simulink model "ddc_bpm_476_066"  (Simulink 7.8)
settings: Solver=ode45  StartTime=0.0  StopTime=4e-4  RelTol=1e-3
undefined symbols (not defined in the file): dt_sim, frev_476, Fs_adc, xlipgetpartsetting
libraries: xbsIndex_r4 x498, simulink x3
(part 2 of 5)

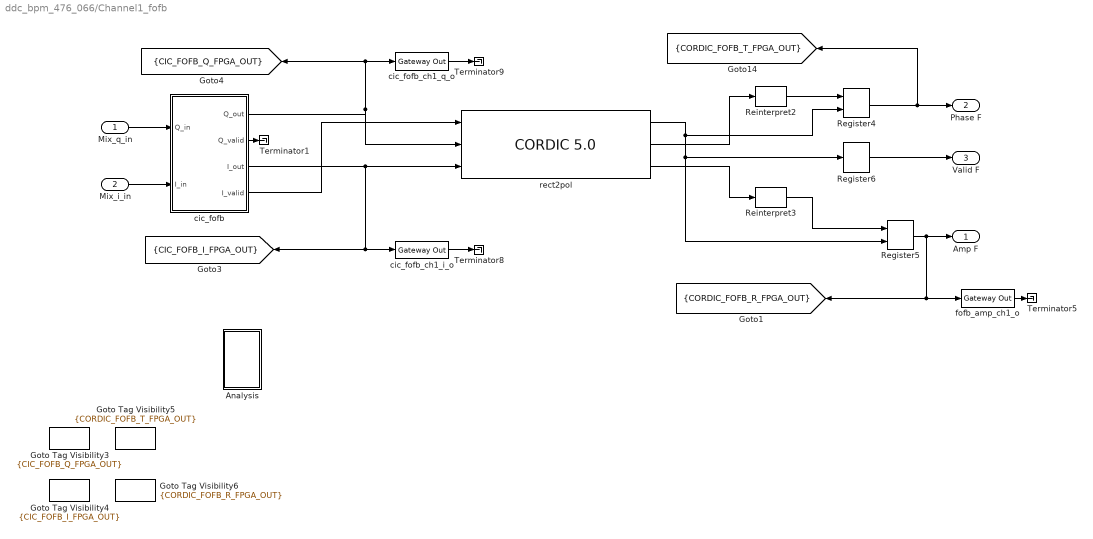
== system ddc_bpm_476_066/Channel1_fofb ==
  Mix_q_in : Inport
  Mix_i_in : Inport  Port=2
  Analysis : Subsystem
  Goto Tag Visibility3 : GotoTagVisibility  GotoTag=CIC_FOFB_Q_FPGA_OUT
  Goto Tag Visibility4 : GotoTagVisibility  GotoTag=CIC_FOFB_I_FPGA_OUT
  Goto Tag Visibility5 : GotoTagVisibility  GotoTag=CORDIC_FOFB_T_FPGA_OUT
  Goto Tag Visibility6 : GotoTagVisibility  GotoTag=CORDIC_FOFB_R_FPGA_OUT
  Register4 : xbsIndex_r4/Register  init=0  rst=off  en=on  dbl_ovrd=off  block_type=register
  Register5 : xbsIndex_r4/Register  init=0  rst=off  en=on  dbl_ovrd=off  block_type=register
  Register6 : xbsIndex_r4/Register  init=0  rst=off  en=off  dbl_ovrd=off  block_type=register
  Reinterpret2 : xbsIndex_r4/Reinterpret  force_arith_type=off  arith_type=Unsigned  force_bin_pt=off  bin_pt=18  block_type=reinterpret
  Reinterpret3 : xbsIndex_r4/Reinterpret  force_arith_type=off  arith_type=Unsigned  force_bin_pt=off  bin_pt=19  block_type=reinterpret
  Terminator{1,5,8..9} (4 alike) : Terminator
  cic_fofb : Subsystem
  cic_fofb_ch1_i_o : xbsIndex_r4/Gateway Out  inherit_from_input=on  hdl_port=on  timing_constraint=Data Rate  locs_specified=off  LOCs={}  UseAsDAC=off  DACChannel='1'  block_type=gatewayout
      settings: infoedit="Gateway out block.  Converts Xilinx fixed-point or floating-point type inputs into ouputs of type Simulink integer, single, double, or fixed point.<br><br>Hardware notes:  In hardware these blocks become top level output ports or are discarded, depending on how they are configured."
  cic_fofb_ch1_q_o : xbsIndex_r4/Gateway Out  inherit_from_input=on  hdl_port=on  timing_constraint=Data Rate  locs_specified=off  LOCs={}  UseAsDAC=off  DACChannel='1'  block_type=gatewayout
      settings: infoedit="Gateway out block.  Converts Xilinx fixed-point or floating-point type inputs into ouputs of type Simulink integer, single, double, or fixed point.<br><br>Hardware notes:  In hardware these blocks become top level output ports or are discarded, depending on how they are configured."
  fofb_amp_ch1_o : xbsIndex_r4/Gateway Out  inherit_from_input=on  hdl_port=on  timing_constraint=Data Rate  locs_specified=off  LOCs={}  UseAsDAC=off  DACChannel='1'  block_type=gatewayout
      settings: infoedit="Gateway out block.  Converts Xilinx fixed-point or floating-point type inputs into ouputs of type Simulink integer, single, double, or fixed point.<br><br>Hardware notes:  In hardware these blocks become top level output ports or are discarded, depending on how they are configured."
  rect2pol : xbsIndex_r4/CORDIC 5.0   functional_selection=Translate  architectural_configuration=Parallel  pipelining_mode=Maximum  data_format=SignedFraction  phase_format=Radians  input_width=25  output_width=25  round_mode=Nearest_Even  iterations=0  precision=0  compensation_scaling=BRAM  coarse_rotation=on  aclken=off  aresetn=off  out_tready=off  cartesian_has_tuser=off  cartesian_has_tlast=off  cartesian_tuser_width=1  phase_has_tuser=off  phase_has_tlast=off  phase_tuser_width=1  out_tlast_behv=Null  flow_control=NonBlocking  optimize_goal=Resources  trim_axipin_name=on  ip_name=CORDIC  ip_version=5.0  dsptool_ready=true  ipcore_usecache=true  ipcore_useipmodelcache=true  wrapper_available=true  port_translation_map={ 'aclken' => 'en', 'aresetn' => 'rst' }  block_type=cordic_v5_0
      settings: infoedit=CORDIC 5.0
  Amp F : Outport
  Phase F : Outport  Port=2
  Valid F : Outport  Port=3
  tag scope: CIC_FOFB_I_FPGA_OUT=scoped, CIC_FOFB_Q_FPGA_OUT=scoped, CORDIC_FOFB_R_FPGA_OUT=scoped, CORDIC_FOFB_T_FPGA_OUT=scoped
  wires:
  cic_fofb/3(I_out) -> rect2pol/3, cic_fofb_ch1_i_o/1, [CIC_FOFB_I_FPGA_OUT]
  cic_fofb/1(Q_out) -> [CIC_FOFB_Q_FPGA_OUT], cic_fofb_ch1_q_o/1, rect2pol/2
  cic_fofb/2(Q_valid) -> Terminator1/1
  rect2pol/1 -> Register4/2, Register5/2, Register6/1
  rect2pol/2 -> Reinterpret2/1
  rect2pol/3 -> Reinterpret3/1
  Register4/1 -> Phase F/1, [CORDIC_FOFB_T_FPGA_OUT]
  Register5/1 -> Amp F/1, [CORDIC_FOFB_R_FPGA_OUT], fofb_amp_ch1_o/1
  Register6/1 -> Valid F/1
  Reinterpret2/1 -> Register4/1
  Reinterpret3/1 -> Register5/1
  fofb_amp_ch1_o/1 -> Terminator5/1
  cic_fofb_ch1_q_o/1 -> Terminator9/1
  cic_fofb_ch1_i_o/1 -> Terminator8/1
  Mix_q_in/1 -> cic_fofb/1(Q_in)
  Mix_i_in/1 -> cic_fofb/2(I_in)
  cic_fofb/4(I_valid) -> rect2pol/1

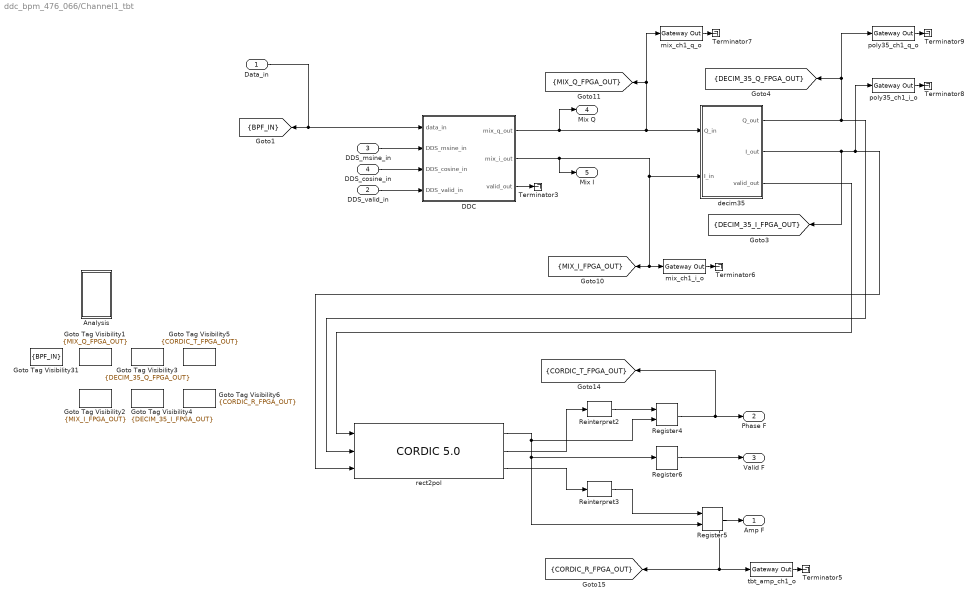
== system ddc_bpm_476_066/Channel1_tbt ==
  Data_in : Inport
  DDS_valid_in : Inport  Port=2
  DDS_msine_in : Inport  Port=3
  DDS_cosine_in : Inport  Port=4
  Analysis : Subsystem
  DDC : Subsystem
  Goto Tag Visibility1 : GotoTagVisibility  GotoTag=MIX_Q_FPGA_OUT
  Goto Tag Visibility2 : GotoTagVisibility  GotoTag=MIX_I_FPGA_OUT
  Goto Tag Visibility3 : GotoTagVisibility  GotoTag=DECIM_35_Q_FPGA_OUT
  Goto Tag Visibility31 : GotoTagVisibility  GotoTag=BPF_IN
  Goto Tag Visibility4 : GotoTagVisibility  GotoTag=DECIM_35_I_FPGA_OUT
  Goto Tag Visibility5 : GotoTagVisibility  GotoTag=CORDIC_T_FPGA_OUT
  Goto Tag Visibility6 : GotoTagVisibility  GotoTag=CORDIC_R_FPGA_OUT
  Register4 : xbsIndex_r4/Register  init=0  rst=off  en=on  dbl_ovrd=off  block_type=register
  Register5 : xbsIndex_r4/Register  init=0  rst=off  en=on  dbl_ovrd=off  block_type=register
  Register6 : xbsIndex_r4/Register  init=0  rst=off  en=off  dbl_ovrd=off  block_type=register
  Reinterpret2 : xbsIndex_r4/Reinterpret  force_arith_type=off  arith_type=Unsigned  force_bin_pt=off  bin_pt=18  block_type=reinterpret
  Reinterpret3 : xbsIndex_r4/Reinterpret  force_arith_type=off  arith_type=Unsigned  force_bin_pt=off  bin_pt=19  block_type=reinterpret
  Terminator{3,5..9} (6 alike) : Terminator
  decim35 : Subsystem
  mix_ch1_i_o : xbsIndex_r4/Gateway Out  inherit_from_input=on  hdl_port=on  timing_constraint=Data Rate  locs_specified=off  LOCs={}  UseAsDAC=off  DACChannel='1'  block_type=gatewayout
      settings: infoedit="Gateway out block.  Converts Xilinx fixed-point or floating-point type inputs into ouputs of type Simulink integer, single, double, or fixed point.<br><br>Hardware notes:  In hardware these blocks become top level output ports or are discarded, depending on how they are configured."
  mix_ch1_q_o : xbsIndex_r4/Gateway Out  inherit_from_input=on  hdl_port=on  timing_constraint=Data Rate  locs_specified=off  LOCs={}  UseAsDAC=off  DACChannel='1'  block_type=gatewayout
      settings: infoedit="Gateway out block.  Converts Xilinx fixed-point or floating-point type inputs into ouputs of type Simulink integer, single, double, or fixed point.<br><br>Hardware notes:  In hardware these blocks become top level output ports or are discarded, depending on how they are configured."
  poly35_ch1_i_o : xbsIndex_r4/Gateway Out  inherit_from_input=on  hdl_port=on  timing_constraint=Data Rate  locs_specified=off  LOCs={}  UseAsDAC=off  DACChannel='1'  block_type=gatewayout
      settings: infoedit="Gateway out block.  Converts Xilinx fixed-point or floating-point type inputs into ouputs of type Simulink integer, single, double, or fixed point.<br><br>Hardware notes:  In hardware these blocks become top level output ports or are discarded, depending on how they are configured."
  poly35_ch1_q_o : xbsIndex_r4/Gateway Out  inherit_from_input=on  hdl_port=on  timing_constraint=Data Rate  locs_specified=off  LOCs={}  UseAsDAC=off  DACChannel='1'  block_type=gatewayout
      settings: infoedit="Gateway out block.  Converts Xilinx fixed-point or floating-point type inputs into ouputs of type Simulink integer, single, double, or fixed point.<br><br>Hardware notes:  In hardware these blocks become top level output ports or are discarded, depending on how they are configured."
  rect2pol : xbsIndex_r4/CORDIC 5.0   functional_selection=Translate  architectural_configuration=Parallel  pipelining_mode=Maximum  data_format=SignedFraction  phase_format=Radians  input_width=25  output_width=25  round_mode=Nearest_Even  iterations=0  precision=0  compensation_scaling=BRAM  coarse_rotation=on  aclken=off  aresetn=off  out_tready=off  cartesian_has_tuser=off  cartesian_has_tlast=off  cartesian_tuser_width=1  phase_has_tuser=off  phase_has_tlast=off  phase_tuser_width=1  out_tlast_behv=Null  flow_control=NonBlocking  optimize_goal=Resources  trim_axipin_name=on  ip_name=CORDIC  ip_version=5.0  dsptool_ready=true  ipcore_usecache=true  ipcore_useipmodelcache=true  wrapper_available=true  port_translation_map={ 'aclken' => 'en', 'aresetn' => 'rst' }  block_type=cordic_v5_0
      settings: infoedit=CORDIC 5.0
  tbt_amp_ch1_o : xbsIndex_r4/Gateway Out  inherit_from_input=on  hdl_port=on  timing_constraint=Data Rate  locs_specified=off  LOCs={}  UseAsDAC=off  DACChannel='1'  block_type=gatewayout
      settings: infoedit="Gateway out block.  Converts Xilinx fixed-point or floating-point type inputs into ouputs of type Simulink integer, single, double, or fixed point.<br><br>Hardware notes:  In hardware these blocks become top level output ports or are discarded, depending on how they are configured."
  Amp F : Outport
  Phase F : Outport  Port=2
  Valid F : Outport  Port=3
  Mix Q : Outport  Port=4
  Mix I : Outport  Port=5
  tag scope: BPF_IN=scoped, CORDIC_R_FPGA_OUT=scoped, CORDIC_T_FPGA_OUT=scoped, DECIM_35_I_FPGA_OUT=scoped, DECIM_35_Q_FPGA_OUT=scoped, MIX_I_FPGA_OUT=scoped, MIX_Q_FPGA_OUT=scoped
  wires:
  Data_in/1 -> [BPF_IN], DDC/1(data_in)
  DDC/2(mix_i_out) -> decim35/2(I_in), [MIX_I_FPGA_OUT], mix_ch1_i_o/1, Mix I/1
  DDC/3(valid_out) -> Terminator3/1
  DDC/1(mix_q_out) -> decim35/1(Q_in), [MIX_Q_FPGA_OUT], mix_ch1_q_o/1, Mix Q/1
  decim35/2(I_out) -> [DECIM_35_I_FPGA_OUT], rect2pol/3, poly35_ch1_i_o/1
  decim35/1(Q_out) -> rect2pol/2, [DECIM_35_Q_FPGA_OUT], poly35_ch1_q_o/1
  decim35/3(valid_out) -> rect2pol/1
  rect2pol/1 -> Register4/2, Register5/2, Register6/1
  rect2pol/2 -> Reinterpret2/1
  rect2pol/3 -> Reinterpret3/1
  Register4/1 -> Phase F/1, [CORDIC_T_FPGA_OUT]
  Register5/1 -> Amp F/1, [CORDIC_R_FPGA_OUT], tbt_amp_ch1_o/1
  Register6/1 -> Valid F/1
  Reinterpret2/1 -> Register4/1
  Reinterpret3/1 -> Register5/1
  tbt_amp_ch1_o/1 -> Terminator5/1
  mix_ch1_i_o/1 -> Terminator6/1
  mix_ch1_q_o/1 -> Terminator7/1
  poly35_ch1_q_o/1 -> Terminator9/1
  poly35_ch1_i_o/1 -> Terminator8/1
  DDS_valid_in/1 -> DDC/4(DDS_valid_in)
  DDS_msine_in/1 -> DDC/2(DDS_msine_in)
  DDS_cosine_in/1 -> DDC/3(DDS_cosine_in)

== system ddc_bpm_476_066/Channel2_fofb ==
  Mix_q_in : Inport
  Mix_i_in : Inport  Port=2
  Analysis : Subsystem
  Goto Tag Visibility3 : GotoTagVisibility  GotoTag=CIC_FOFB_Q_FPGA_OUT
  Goto Tag Visibility4 : GotoTagVisibility  GotoTag=CIC_FOFB_I_FPGA_OUT
  Goto Tag Visibility5 : GotoTagVisibility  GotoTag=CORDIC_FOFB_T_FPGA_OUT
  Goto Tag Visibility6 : GotoTagVisibility  GotoTag=CORDIC_FOFB_R_FPGA_OUT
  Register4 : xbsIndex_r4/Register  init=0  rst=off  en=on  dbl_ovrd=off  block_type=register
  Register5 : xbsIndex_r4/Register  init=0  rst=off  en=on  dbl_ovrd=off  block_type=register
  Register6 : xbsIndex_r4/Register  init=0  rst=off  en=off  dbl_ovrd=off  block_type=register
  Reinterpret2 : xbsIndex_r4/Reinterpret  force_arith_type=off  arith_type=Unsigned  force_bin_pt=off  bin_pt=18  block_type=reinterpret
  Reinterpret3 : xbsIndex_r4/Reinterpret  force_arith_type=off  arith_type=Unsigned  force_bin_pt=off  bin_pt=19  block_type=reinterpret
  Terminator{1,5,8..9} (4 alike) : Terminator
  cic_fofb : Subsystem
  cic_fofb_ch2_i_o : xbsIndex_r4/Gateway Out  inherit_from_input=on  hdl_port=on  timing_constraint=Data Rate  locs_specified=off  LOCs={}  UseAsDAC=off  DACChannel='1'  block_type=gatewayout
      settings: infoedit="Gateway out block.  Converts Xilinx fixed-point or floating-point type inputs into ouputs of type Simulink integer, single, double, or fixed point.<br><br>Hardware notes:  In hardware these blocks become top level output ports or are discarded, depending on how they are configured."
  cic_fofb_ch2_q_o : xbsIndex_r4/Gateway Out  inherit_from_input=on  hdl_port=on  timing_constraint=Data Rate  locs_specified=off  LOCs={}  UseAsDAC=off  DACChannel='1'  block_type=gatewayout
      settings: infoedit="Gateway out block.  Converts Xilinx fixed-point or floating-point type inputs into ouputs of type Simulink integer, single, double, or fixed point.<br><br>Hardware notes:  In hardware these blocks become top level output ports or are discarded, depending on how they are configured."
  fofb_amp_ch2_o : xbsIndex_r4/Gateway Out  inherit_from_input=on  hdl_port=on  timing_constraint=Data Rate  locs_specified=off  LOCs={}  UseAsDAC=off  DACChannel='1'  block_type=gatewayout
      settings: infoedit="Gateway out block.  Converts Xilinx fixed-point or floating-point type inputs into ouputs of type Simulink integer, single, double, or fixed point.<br><br>Hardware notes:  In hardware these blocks become top level output ports or are discarded, depending on how they are configured."
  rect2pol : xbsIndex_r4/CORDIC 5.0   functional_selection=Translate  architectural_configuration=Parallel  pipelining_mode=Maximum  data_format=SignedFraction  phase_format=Radians  input_width=25  output_width=25  round_mode=Nearest_Even  iterations=0  precision=0  compensation_scaling=BRAM  coarse_rotation=on  aclken=off  aresetn=off  out_tready=off  cartesian_has_tuser=off  cartesian_has_tlast=off  cartesian_tuser_width=1  phase_has_tuser=off  phase_has_tlast=off  phase_tuser_width=1  out_tlast_behv=Null  flow_control=NonBlocking  optimize_goal=Resources  trim_axipin_name=on  ip_name=CORDIC  ip_version=5.0  dsptool_ready=true  ipcore_usecache=true  ipcore_useipmodelcache=true  wrapper_available=true  port_translation_map={ 'aclken' => 'en', 'aresetn' => 'rst' }  block_type=cordic_v5_0
      settings: infoedit=CORDIC 5.0
  Amp F : Outport
  Phase F : Outport  Port=2
  Valid F : Outport  Port=3
  tag scope: CIC_FOFB_I_FPGA_OUT=scoped, CIC_FOFB_Q_FPGA_OUT=scoped, CORDIC_FOFB_R_FPGA_OUT=scoped, CORDIC_FOFB_T_FPGA_OUT=scoped
  wires:
  cic_fofb/3(I_out) -> rect2pol/3, cic_fofb_ch2_i_o/1, [CIC_FOFB_I_FPGA_OUT]
  cic_fofb/1(Q_out) -> [CIC_FOFB_Q_FPGA_OUT], cic_fofb_ch2_q_o/1, rect2pol/2
  cic_fofb/2(Q_valid) -> Terminator1/1
  rect2pol/1 -> Register4/2, Register5/2, Register6/1
  rect2pol/2 -> Reinterpret2/1
  rect2pol/3 -> Reinterpret3/1
  Register4/1 -> Phase F/1, [CORDIC_FOFB_T_FPGA_OUT]
  Register5/1 -> Amp F/1, [CORDIC_FOFB_R_FPGA_OUT], fofb_amp_ch2_o/1
  Register6/1 -> Valid F/1
  Reinterpret2/1 -> Register4/1
  Reinterpret3/1 -> Register5/1
  fofb_amp_ch2_o/1 -> Terminator5/1
  cic_fofb_ch2_q_o/1 -> Terminator9/1
  cic_fofb_ch2_i_o/1 -> Terminator8/1
  Mix_q_in/1 -> cic_fofb/1(Q_in)
  Mix_i_in/1 -> cic_fofb/2(I_in)
  cic_fofb/4(I_valid) -> rect2pol/1

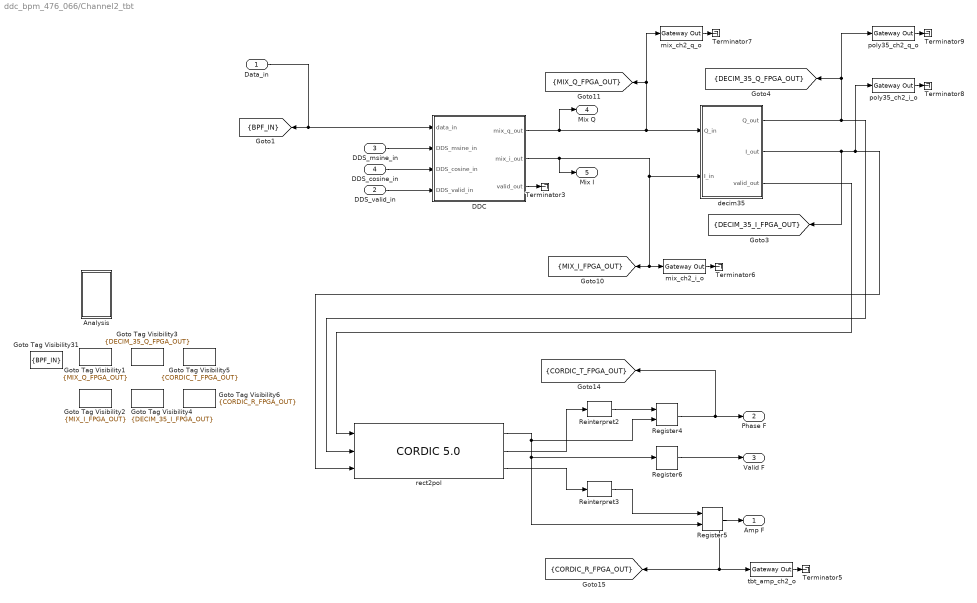
== system ddc_bpm_476_066/Channel2_tbt ==
  Data_in : Inport
  DDS_valid_in : Inport  Port=2
  DDS_msine_in : Inport  Port=3
  DDS_cosine_in : Inport  Port=4
  Analysis : Subsystem
  DDC : Subsystem
  Goto Tag Visibility1 : GotoTagVisibility  GotoTag=MIX_Q_FPGA_OUT
  Goto Tag Visibility2 : GotoTagVisibility  GotoTag=MIX_I_FPGA_OUT
  Goto Tag Visibility3 : GotoTagVisibility  GotoTag=DECIM_35_Q_FPGA_OUT
  Goto Tag Visibility31 : GotoTagVisibility  GotoTag=BPF_IN
  Goto Tag Visibility4 : GotoTagVisibility  GotoTag=DECIM_35_I_FPGA_OUT
  Goto Tag Visibility5 : GotoTagVisibility  GotoTag=CORDIC_T_FPGA_OUT
  Goto Tag Visibility6 : GotoTagVisibility  GotoTag=CORDIC_R_FPGA_OUT
  Register4 : xbsIndex_r4/Register  init=0  rst=off  en=on  dbl_ovrd=off  block_type=register
  Register5 : xbsIndex_r4/Register  init=0  rst=off  en=on  dbl_ovrd=off  block_type=register
  Register6 : xbsIndex_r4/Register  init=0  rst=off  en=off  dbl_ovrd=off  block_type=register
  Reinterpret2 : xbsIndex_r4/Reinterpret  force_arith_type=off  arith_type=Unsigned  force_bin_pt=off  bin_pt=18  block_type=reinterpret
  Reinterpret3 : xbsIndex_r4/Reinterpret  force_arith_type=off  arith_type=Unsigned  force_bin_pt=off  bin_pt=19  block_type=reinterpret
  Terminator{3,5..9} (6 alike) : Terminator
  decim35 : Subsystem
  mix_ch2_i_o : xbsIndex_r4/Gateway Out  inherit_from_input=on  hdl_port=on  timing_constraint=Data Rate  locs_specified=off  LOCs={}  UseAsDAC=off  DACChannel='1'  block_type=gatewayout
      settings: infoedit="Gateway out block.  Converts Xilinx fixed-point or floating-point type inputs into ouputs of type Simulink integer, single, double, or fixed point.<br><br>Hardware notes:  In hardware these blocks become top level output ports or are discarded, depending on how they are configured."
  mix_ch2_q_o : xbsIndex_r4/Gateway Out  inherit_from_input=on  hdl_port=on  timing_constraint=Data Rate  locs_specified=off  LOCs={}  UseAsDAC=off  DACChannel='1'  block_type=gatewayout
      settings: infoedit="Gateway out block.  Converts Xilinx fixed-point or floating-point type inputs into ouputs of type Simulink integer, single, double, or fixed point.<br><br>Hardware notes:  In hardware these blocks become top level output ports or are discarded, depending on how they are configured."
  poly35_ch2_i_o : xbsIndex_r4/Gateway Out  inherit_from_input=on  hdl_port=on  timing_constraint=Data Rate  locs_specified=off  LOCs={}  UseAsDAC=off  DACChannel='1'  block_type=gatewayout
      settings: infoedit="Gateway out block.  Converts Xilinx fixed-point or floating-point type inputs into ouputs of type Simulink integer, single, double, or fixed point.<br><br>Hardware notes:  In hardware these blocks become top level output ports or are discarded, depending on how they are configured."
  poly35_ch2_q_o : xbsIndex_r4/Gateway Out  inherit_from_input=on  hdl_port=on  timing_constraint=Data Rate  locs_specified=off  LOCs={}  UseAsDAC=off  DACChannel='1'  block_type=gatewayout
      settings: infoedit="Gateway out block.  Converts Xilinx fixed-point or floating-point type inputs into ouputs of type Simulink integer, single, double, or fixed point.<br><br>Hardware notes:  In hardware these blocks become top level output ports or are discarded, depending on how they are configured."
  rect2pol : xbsIndex_r4/CORDIC 5.0   functional_selection=Translate  architectural_configuration=Parallel  pipelining_mode=Maximum  data_format=SignedFraction  phase_format=Radians  input_width=25  output_width=25  round_mode=Nearest_Even  iterations=0  precision=0  compensation_scaling=BRAM  coarse_rotation=on  aclken=off  aresetn=off  out_tready=off  cartesian_has_tuser=off  cartesian_has_tlast=off  cartesian_tuser_width=1  phase_has_tuser=off  phase_has_tlast=off  phase_tuser_width=1  out_tlast_behv=Null  flow_control=NonBlocking  optimize_goal=Resources  trim_axipin_name=on  ip_name=CORDIC  ip_version=5.0  dsptool_ready=true  ipcore_usecache=true  ipcore_useipmodelcache=true  wrapper_available=true  port_translation_map={ 'aclken' => 'en', 'aresetn' => 'rst' }  block_type=cordic_v5_0
      settings: infoedit=CORDIC 5.0
  tbt_amp_ch2_o : xbsIndex_r4/Gateway Out  inherit_from_input=on  hdl_port=on  timing_constraint=Data Rate  locs_specified=off  LOCs={}  UseAsDAC=off  DACChannel='1'  block_type=gatewayout
      settings: infoedit="Gateway out block.  Converts Xilinx fixed-point or floating-point type inputs into ouputs of type Simulink integer, single, double, or fixed point.<br><br>Hardware notes:  In hardware these blocks become top level output ports or are discarded, depending on how they are configured."
  Amp F : Outport
  Phase F : Outport  Port=2
  Valid F : Outport  Port=3
  Mix Q : Outport  Port=4
  Mix I : Outport  Port=5
  tag scope: BPF_IN=scoped, CORDIC_R_FPGA_OUT=scoped, CORDIC_T_FPGA_OUT=scoped, DECIM_35_I_FPGA_OUT=scoped, DECIM_35_Q_FPGA_OUT=scoped, MIX_I_FPGA_OUT=scoped, MIX_Q_FPGA_OUT=scoped
  wires:
  Data_in/1 -> [BPF_IN], DDC/1(data_in)
  DDC/2(mix_i_out) -> decim35/2(I_in), [MIX_I_FPGA_OUT], mix_ch2_i_o/1, Mix I/1
  DDC/3(valid_out) -> Terminator3/1
  DDC/1(mix_q_out) -> decim35/1(Q_in), [MIX_Q_FPGA_OUT], mix_ch2_q_o/1, Mix Q/1
  decim35/2(I_out) -> [DECIM_35_I_FPGA_OUT], rect2pol/3, poly35_ch2_i_o/1
  decim35/1(Q_out) -> rect2pol/2, [DECIM_35_Q_FPGA_OUT], poly35_ch2_q_o/1
  decim35/3(valid_out) -> rect2pol/1
  rect2pol/1 -> Register4/2, Register5/2, Register6/1
  rect2pol/2 -> Reinterpret2/1
  rect2pol/3 -> Reinterpret3/1
  Register4/1 -> Phase F/1, [CORDIC_T_FPGA_OUT]
  Register5/1 -> Amp F/1, [CORDIC_R_FPGA_OUT], tbt_amp_ch2_o/1
  Register6/1 -> Valid F/1
  Reinterpret2/1 -> Register4/1
  Reinterpret3/1 -> Register5/1
  tbt_amp_ch2_o/1 -> Terminator5/1
  mix_ch2_i_o/1 -> Terminator6/1
  mix_ch2_q_o/1 -> Terminator7/1
  poly35_ch2_q_o/1 -> Terminator9/1
  poly35_ch2_i_o/1 -> Terminator8/1
  DDS_valid_in/1 -> DDC/4(DDS_valid_in)
  DDS_msine_in/1 -> DDC/2(DDS_msine_in)
  DDS_cosine_in/1 -> DDC/3(DDS_cosine_in)

== system ddc_bpm_476_066/Channel3_fofb ==
  Mix_q_in : Inport
  Mix_i_in : Inport  Port=2
  Analysis : Subsystem
  Goto Tag Visibility3 : GotoTagVisibility  GotoTag=CIC_FOFB_Q_FPGA_OUT
  Goto Tag Visibility4 : GotoTagVisibility  GotoTag=CIC_FOFB_I_FPGA_OUT
  Goto Tag Visibility5 : GotoTagVisibility  GotoTag=CORDIC_FOFB_T_FPGA_OUT
  Goto Tag Visibility6 : GotoTagVisibility  GotoTag=CORDIC_FOFB_R_FPGA_OUT
  Register4 : xbsIndex_r4/Register  init=0  rst=off  en=on  dbl_ovrd=off  block_type=register
  Register5 : xbsIndex_r4/Register  init=0  rst=off  en=on  dbl_ovrd=off  block_type=register
  Register6 : xbsIndex_r4/Register  init=0  rst=off  en=off  dbl_ovrd=off  block_type=register
  Reinterpret2 : xbsIndex_r4/Reinterpret  force_arith_type=off  arith_type=Unsigned  force_bin_pt=off  bin_pt=18  block_type=reinterpret
  Reinterpret3 : xbsIndex_r4/Reinterpret  force_arith_type=off  arith_type=Unsigned  force_bin_pt=off  bin_pt=19  block_type=reinterpret
  Terminator{1,5,8..9} (4 alike) : Terminator
  cic_fofb : Subsystem
  cic_fofb_ch3_i_o : xbsIndex_r4/Gateway Out  inherit_from_input=on  hdl_port=on  timing_constraint=Data Rate  locs_specified=off  LOCs={}  UseAsDAC=off  DACChannel='1'  block_type=gatewayout
      settings: infoedit="Gateway out block.  Converts Xilinx fixed-point or floating-point type inputs into ouputs of type Simulink integer, single, double, or fixed point.<br><br>Hardware notes:  In hardware these blocks become top level output ports or are discarded, depending on how they are configured."
  cic_fofb_ch3_q_o : xbsIndex_r4/Gateway Out  inherit_from_input=on  hdl_port=on  timing_constraint=Data Rate  locs_specified=off  LOCs={}  UseAsDAC=off  DACChannel='1'  block_type=gatewayout
      settings: infoedit="Gateway out block.  Converts Xilinx fixed-point or floating-point type inputs into ouputs of type Simulink integer, single, double, or fixed point.<br><br>Hardware notes:  In hardware these blocks become top level output ports or are discarded, depending on how they are configured."
  fofb_amp_ch3_o : xbsIndex_r4/Gateway Out  inherit_from_input=on  hdl_port=on  timing_constraint=Data Rate  locs_specified=off  LOCs={}  UseAsDAC=off  DACChannel='1'  block_type=gatewayout
      settings: infoedit="Gateway out block.  Converts Xilinx fixed-point or floating-point type inputs into ouputs of type Simulink integer, single, double, or fixed point.<br><br>Hardware notes:  In hardware these blocks become top level output ports or are discarded, depending on how they are configured."
  rect2pol : xbsIndex_r4/CORDIC 5.0   functional_selection=Translate  architectural_configuration=Parallel  pipelining_mode=Maximum  data_format=SignedFraction  phase_format=Radians  input_width=25  output_width=25  round_mode=Nearest_Even  iterations=0  precision=0  compensation_scaling=BRAM  coarse_rotation=on  aclken=off  aresetn=off  out_tready=off  cartesian_has_tuser=off  cartesian_has_tlast=off  cartesian_tuser_width=1  phase_has_tuser=off  phase_has_tlast=off  phase_tuser_width=1  out_tlast_behv=Null  flow_control=NonBlocking  optimize_goal=Resources  trim_axipin_name=on  ip_name=CORDIC  ip_version=5.0  dsptool_ready=true  ipcore_usecache=true  ipcore_useipmodelcache=true  wrapper_available=true  port_translation_map={ 'aclken' => 'en', 'aresetn' => 'rst' }  block_type=cordic_v5_0
      settings: infoedit=CORDIC 5.0
  Amp F : Outport
  Phase F : Outport  Port=2
  Valid F : Outport  Port=3
  tag scope: CIC_FOFB_I_FPGA_OUT=scoped, CIC_FOFB_Q_FPGA_OUT=scoped, CORDIC_FOFB_R_FPGA_OUT=scoped, CORDIC_FOFB_T_FPGA_OUT=scoped
  wires:
  cic_fofb/3(I_out) -> rect2pol/3, cic_fofb_ch3_i_o/1, [CIC_FOFB_I_FPGA_OUT]
  cic_fofb/1(Q_out) -> [CIC_FOFB_Q_FPGA_OUT], cic_fofb_ch3_q_o/1, rect2pol/2
  cic_fofb/2(Q_valid) -> Terminator1/1
  rect2pol/1 -> Register4/2, Register5/2, Register6/1
  rect2pol/2 -> Reinterpret2/1
  rect2pol/3 -> Reinterpret3/1
  Register4/1 -> Phase F/1, [CORDIC_FOFB_T_FPGA_OUT]
  Register5/1 -> Amp F/1, [CORDIC_FOFB_R_FPGA_OUT], fofb_amp_ch3_o/1
  Register6/1 -> Valid F/1
  Reinterpret2/1 -> Register4/1
  Reinterpret3/1 -> Register5/1
  fofb_amp_ch3_o/1 -> Terminator5/1
  cic_fofb_ch3_q_o/1 -> Terminator9/1
  cic_fofb_ch3_i_o/1 -> Terminator8/1
  Mix_q_in/1 -> cic_fofb/1(Q_in)
  Mix_i_in/1 -> cic_fofb/2(I_in)
  cic_fofb/4(I_valid) -> rect2pol/1

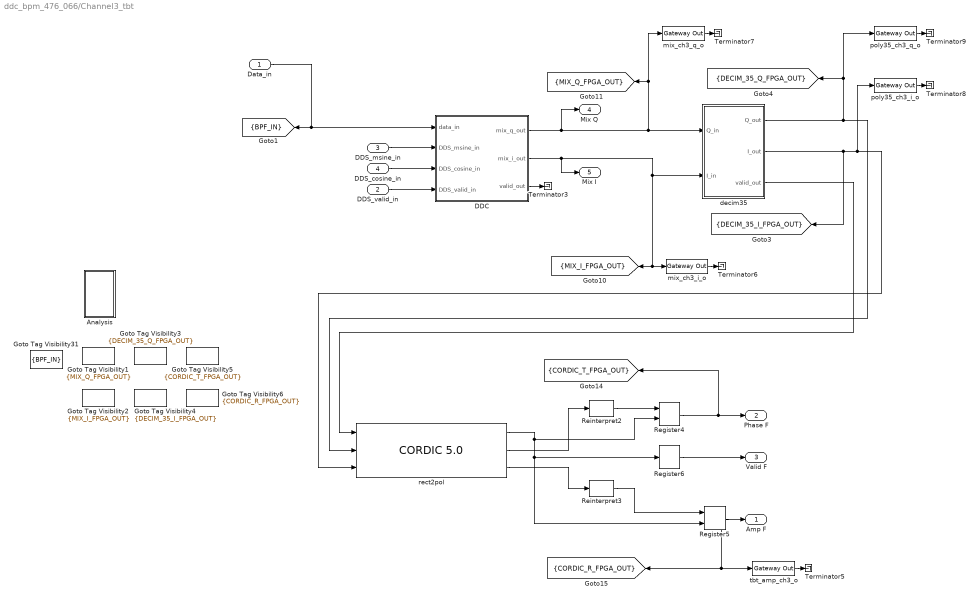
== system ddc_bpm_476_066/Channel3_tbt ==
  Data_in : Inport
  DDS_valid_in : Inport  Port=2
  DDS_msine_in : Inport  Port=3
  DDS_cosine_in : Inport  Port=4
  Analysis : Subsystem
  DDC : Subsystem
  Goto Tag Visibility1 : GotoTagVisibility  GotoTag=MIX_Q_FPGA_OUT
  Goto Tag Visibility2 : GotoTagVisibility  GotoTag=MIX_I_FPGA_OUT
  Goto Tag Visibility3 : GotoTagVisibility  GotoTag=DECIM_35_Q_FPGA_OUT
  Goto Tag Visibility31 : GotoTagVisibility  GotoTag=BPF_IN
  Goto Tag Visibility4 : GotoTagVisibility  GotoTag=DECIM_35_I_FPGA_OUT
  Goto Tag Visibility5 : GotoTagVisibility  GotoTag=CORDIC_T_FPGA_OUT
  Goto Tag Visibility6 : GotoTagVisibility  GotoTag=CORDIC_R_FPGA_OUT
  Register4 : xbsIndex_r4/Register  init=0  rst=off  en=on  dbl_ovrd=off  block_type=register
  Register5 : xbsIndex_r4/Register  init=0  rst=off  en=on  dbl_ovrd=off  block_type=register
  Register6 : xbsIndex_r4/Register  init=0  rst=off  en=off  dbl_ovrd=off  block_type=register
  Reinterpret2 : xbsIndex_r4/Reinterpret  force_arith_type=off  arith_type=Unsigned  force_bin_pt=off  bin_pt=18  block_type=reinterpret
  Reinterpret3 : xbsIndex_r4/Reinterpret  force_arith_type=off  arith_type=Unsigned  force_bin_pt=off  bin_pt=19  block_type=reinterpret
  Terminator{3,5..9} (6 alike) : Terminator
  decim35 : Subsystem
  mix_ch3_i_o : xbsIndex_r4/Gateway Out  inherit_from_input=on  hdl_port=on  timing_constraint=Data Rate  locs_specified=off  LOCs={}  UseAsDAC=off  DACChannel='1'  block_type=gatewayout
      settings: infoedit="Gateway out block.  Converts Xilinx fixed-point or floating-point type inputs into ouputs of type Simulink integer, single, double, or fixed point.<br><br>Hardware notes:  In hardware these blocks become top level output ports or are discarded, depending on how they are configured."
  mix_ch3_q_o : xbsIndex_r4/Gateway Out  inherit_from_input=on  hdl_port=on  timing_constraint=Data Rate  locs_specified=off  LOCs={}  UseAsDAC=off  DACChannel='1'  block_type=gatewayout
      settings: infoedit="Gateway out block.  Converts Xilinx fixed-point or floating-point type inputs into ouputs of type Simulink integer, single, double, or fixed point.<br><br>Hardware notes:  In hardware these blocks become top level output ports or are discarded, depending on how they are configured."
  poly35_ch3_i_o : xbsIndex_r4/Gateway Out  inherit_from_input=on  hdl_port=on  timing_constraint=Data Rate  locs_specified=off  LOCs={}  UseAsDAC=off  DACChannel='1'  block_type=gatewayout
      settings: infoedit="Gateway out block.  Converts Xilinx fixed-point or floating-point type inputs into ouputs of type Simulink integer, single, double, or fixed point.<br><br>Hardware notes:  In hardware these blocks become top level output ports or are discarded, depending on how they are configured."
  poly35_ch3_q_o : xbsIndex_r4/Gateway Out  inherit_from_input=on  hdl_port=on  timing_constraint=Data Rate  locs_specified=off  LOCs={}  UseAsDAC=off  DACChannel='1'  block_type=gatewayout
      settings: infoedit="Gateway out block.  Converts Xilinx fixed-point or floating-point type inputs into ouputs of type Simulink integer, single, double, or fixed point.<br><br>Hardware notes:  In hardware these blocks become top level output ports or are discarded, depending on how they are configured."
  rect2pol : xbsIndex_r4/CORDIC 5.0   functional_selection=Translate  architectural_configuration=Parallel  pipelining_mode=Maximum  data_format=SignedFraction  phase_format=Radians  input_width=25  output_width=25  round_mode=Nearest_Even  iterations=0  precision=0  compensation_scaling=BRAM  coarse_rotation=on  aclken=off  aresetn=off  out_tready=off  cartesian_has_tuser=off  cartesian_has_tlast=off  cartesian_tuser_width=1  phase_has_tuser=off  phase_has_tlast=off  phase_tuser_width=1  out_tlast_behv=Null  flow_control=NonBlocking  optimize_goal=Resources  trim_axipin_name=on  ip_name=CORDIC  ip_version=5.0  dsptool_ready=true  ipcore_usecache=true  ipcore_useipmodelcache=true  wrapper_available=true  port_translation_map={ 'aclken' => 'en', 'aresetn' => 'rst' }  block_type=cordic_v5_0
      settings: infoedit=CORDIC 5.0
  tbt_amp_ch3_o : xbsIndex_r4/Gateway Out  inherit_from_input=on  hdl_port=on  timing_constraint=Data Rate  locs_specified=off  LOCs={}  UseAsDAC=off  DACChannel='1'  block_type=gatewayout
      settings: infoedit="Gateway out block.  Converts Xilinx fixed-point or floating-point type inputs into ouputs of type Simulink integer, single, double, or fixed point.<br><br>Hardware notes:  In hardware these blocks become top level output ports or are discarded, depending on how they are configured."
  Amp F : Outport
  Phase F : Outport  Port=2
  Valid F : Outport  Port=3
  Mix Q : Outport  Port=4
  Mix I : Outport  Port=5
  tag scope: BPF_IN=scoped, CORDIC_R_FPGA_OUT=scoped, CORDIC_T_FPGA_OUT=scoped, DECIM_35_I_FPGA_OUT=scoped, DECIM_35_Q_FPGA_OUT=scoped, MIX_I_FPGA_OUT=scoped, MIX_Q_FPGA_OUT=scoped
  wires:
  Data_in/1 -> [BPF_IN], DDC/1(data_in)
  DDC/2(mix_i_out) -> decim35/2(I_in), [MIX_I_FPGA_OUT], mix_ch3_i_o/1, Mix I/1
  DDC/3(valid_out) -> Terminator3/1
  DDC/1(mix_q_out) -> decim35/1(Q_in), [MIX_Q_FPGA_OUT], mix_ch3_q_o/1, Mix Q/1
  decim35/2(I_out) -> [DECIM_35_I_FPGA_OUT], rect2pol/3, poly35_ch3_i_o/1
  decim35/1(Q_out) -> rect2pol/2, [DECIM_35_Q_FPGA_OUT], poly35_ch3_q_o/1
  decim35/3(valid_out) -> rect2pol/1
  rect2pol/1 -> Register4/2, Register5/2, Register6/1
  rect2pol/2 -> Reinterpret2/1
  rect2pol/3 -> Reinterpret3/1
  Register4/1 -> Phase F/1, [CORDIC_T_FPGA_OUT]
  Register5/1 -> Amp F/1, [CORDIC_R_FPGA_OUT], tbt_amp_ch3_o/1
  Register6/1 -> Valid F/1
  Reinterpret2/1 -> Register4/1
  Reinterpret3/1 -> Register5/1
  tbt_amp_ch3_o/1 -> Terminator5/1
  mix_ch3_i_o/1 -> Terminator6/1
  mix_ch3_q_o/1 -> Terminator7/1
  poly35_ch3_q_o/1 -> Terminator9/1
  poly35_ch3_i_o/1 -> Terminator8/1
  DDS_valid_in/1 -> DDC/4(DDS_valid_in)
  DDS_msine_in/1 -> DDC/2(DDS_msine_in)
  DDS_cosine_in/1 -> DDC/3(DDS_cosine_in)

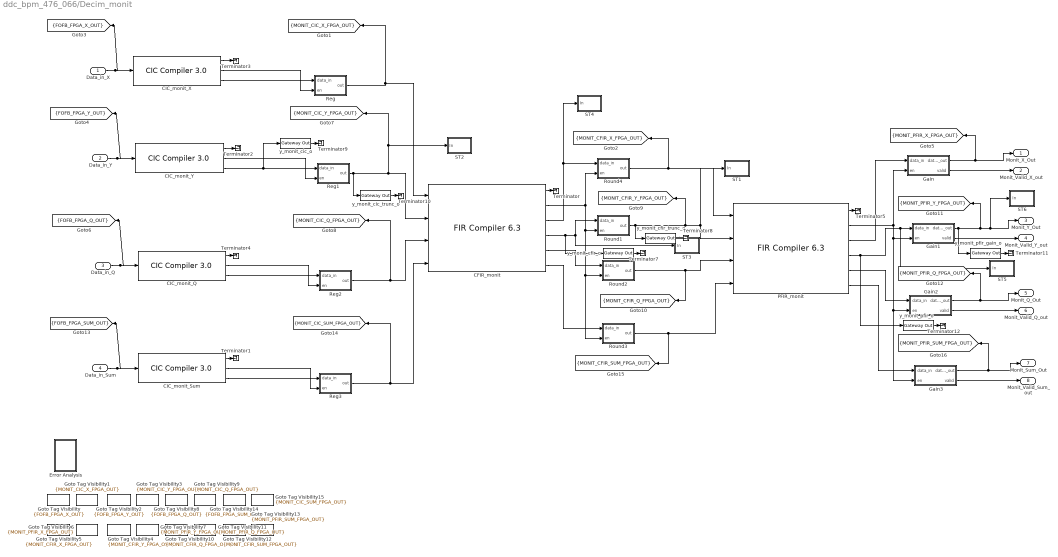
== system ddc_bpm_476_066/Decim_monit ==
  Data_in_X : Inport
  Data_in_Y : Inport  Port=2
  Data_in_Q : Inport  Port=3
  Data_in_Sum : Inport  Port=4
  CFIR_monit : xbsIndex_r4/FIR Compiler 6.3   coefficientvector=hcfir_sec.Numerator  coefficient_sets=1  coefficient_reload=off  filter_type=Decimation  rate_change_type=Integer  interpolation_rate=1  decimation_rate=2  zero_pack_factor=1  channel_sequence=Basic  number_channels=1  pattern_list='P4-0,P4-1,P4-2,P4-3,P4-4'  number_paths=4  ratespecification=Hardware_Oversampling_Rate  sampleperiod=5565000  hardwareoversamplingrate=1  coefficient_sign=Signed  quantization=Integer_Coefficients  coefficient_width=16  bestprecision=off  coefficient_fractional_bits=0  coefficient_structure=Inferred  output_rounding_mode=Full_Precision  output_width=36  filter_architecture=Systolic_Multiply_Accumulate  optimization_goal=Area  data_buffer_type=Automatic  coefficient_buffer_type=Automatic  input_buffer_type=Automatic  output_buffer_type=Automatic  preference_for_other_storage=Automatic  multi_column_support=Automatic  columnconfig='8'  inter_column_pipe_length=4  data_has_tlast=Not_Required  m_data_has_tready=off  s_data_has_fifo=off  s_data_has_tuser=Not_Required  m_data_has_tuser=Not_Required  s_config_sync_mode=On_Vector  s_config_method=Single  num_reload_slots=1  has_aclken=off  has_aresetn=off  infoeditControl=ARESETn must be asserted for a minmum of 2 cycles  trim_axipin_name=on  passband_min=0.0  passband_max=0.5  stopband_min=0.5  stopband_max=1.0  filter_selection=1  gui_behaviour=Sysgen_GUI  data_sign=Signed  data_width=16  data_fractional_bits=0  data_tuser_width=1  wrapper_available=true  ip_wrap_arbitrary_binary_point=true  simulation_type=external_xfix  simulation_model=firv6_3_CModel:firv6_3_cmodel  ip_name=FIR Compiler  ip_version=6.3  dsptool_ready=true  ipcore_usecache=true  ipcore_useipmodelcache=true  ipcore_xco_need_fpga_part=true  port_translation_map={ 'aclken' => 'en', 'aresetn' => 'rst' }  run_core_at_system_period=true  ipcore_fpga_part=xlipgetpartsetting(gcb, {'virtex6', 'xc6vlx75t', '-3', 'ff784'})  block_type=fir_compiler_v6_3
      settings: infoedit=Maximum Possible : Maximizes oversampling rate. Abstracted input handshake (no s_data_tvalid) and automatic rate propagation.<br>Hardware Oversampling Rate : Specifies oversampling rate relative to the input sample period. Abstracted input handshake (no s_data_tvalid) and automatic rate propagation.<br>Sample Period : Specifies absolute oversampling rate. No input handshake abstraction (exposes s_data_tvalid) and no rate propagation.
  CIC_monit_Q : xbsIndex_r4/CIC Compiler 3.0   filter_type=Decimation  number_of_stages=5  differential_delay=2  number_of_channels=1  sample_rate_changes=Fixed  fixed_or_initial_rate=R_sec  minimum_rate=2500  maximum_rate=2500  ratespecification=Maximum_Possible  sampleperiod=1  hardwareoversamplingrate=1  quantization=Truncation  output_data_width=24  use_xtreme_dsp_slice=on  use_streaming_interface=on  has_aclken=off  has_aresetn=off  has_dout_tready=off  trim_axipin_name=on  gui_behaviour=Sysgen_GUI  input_data_width=18  ip_name=CIC Compiler  ip_version=3.0  dsptool_ready=true  wrapper_available=true  port_translation_map={ 'aclken' => 'en', 'aresetn' => 'rst' }  ipcore_xco_need_fpga_part=true  ipcore_fpga_part=xlipgetpartsetting(gcb, {'virtex7', 'xc7v1500t', '-2', 'fhg1157'})  ipcore_verbose=false  block_type=cic_compiler_v3_0
  CIC_monit_Sum : xbsIndex_r4/CIC Compiler 3.0   filter_type=Decimation  number_of_stages=5  differential_delay=2  number_of_channels=1  sample_rate_changes=Fixed  fixed_or_initial_rate=R_sec  minimum_rate=2500  maximum_rate=2500  ratespecification=Maximum_Possible  sampleperiod=1  hardwareoversamplingrate=1  quantization=Truncation  output_data_width=24  use_xtreme_dsp_slice=on  use_streaming_interface=on  has_aclken=off  has_aresetn=off  has_dout_tready=off  trim_axipin_name=on  gui_behaviour=Sysgen_GUI  input_data_width=18  ip_name=CIC Compiler  ip_version=3.0  dsptool_ready=true  wrapper_available=true  port_translation_map={ 'aclken' => 'en', 'aresetn' => 'rst' }  ipcore_xco_need_fpga_part=true  ipcore_fpga_part=xlipgetpartsetting(gcb, {'virtex7', 'xc7v1500t', '-2', 'fhg1157'})  ipcore_verbose=false  block_type=cic_compiler_v3_0
  CIC_monit_X : xbsIndex_r4/CIC Compiler 3.0   filter_type=Decimation  number_of_stages=5  differential_delay=2  number_of_channels=1  sample_rate_changes=Fixed  fixed_or_initial_rate=R_sec  minimum_rate=2500  maximum_rate=2500  ratespecification=Maximum_Possible  sampleperiod=1  hardwareoversamplingrate=1  quantization=Truncation  output_data_width=24  use_xtreme_dsp_slice=on  use_streaming_interface=on  has_aclken=off  has_aresetn=off  has_dout_tready=off  trim_axipin_name=on  gui_behaviour=Sysgen_GUI  input_data_width=18  ip_name=CIC Compiler  ip_version=3.0  dsptool_ready=true  wrapper_available=true  port_translation_map={ 'aclken' => 'en', 'aresetn' => 'rst' }  ipcore_xco_need_fpga_part=true  ipcore_fpga_part=xlipgetpartsetting(gcb, {'virtex7', 'xc7v1500t', '-2', 'fhg1157'})  ipcore_verbose=false  block_type=cic_compiler_v3_0
  CIC_monit_Y : xbsIndex_r4/CIC Compiler 3.0   filter_type=Decimation  number_of_stages=5  differential_delay=2  number_of_channels=1  sample_rate_changes=Fixed  fixed_or_initial_rate=R_sec  minimum_rate=2500  maximum_rate=2500  ratespecification=Maximum_Possible  sampleperiod=1  hardwareoversamplingrate=1  quantization=Truncation  output_data_width=24  use_xtreme_dsp_slice=on  use_streaming_interface=on  has_aclken=off  has_aresetn=off  has_dout_tready=off  trim_axipin_name=on  gui_behaviour=Sysgen_GUI  input_data_width=18  ip_name=CIC Compiler  ip_version=3.0  dsptool_ready=true  wrapper_available=true  port_translation_map={ 'aclken' => 'en', 'aresetn' => 'rst' }  ipcore_xco_need_fpga_part=true  ipcore_fpga_part=xlipgetpartsetting(gcb, {'virtex7', 'xc7v1500t', '-2', 'fhg1157'})  ipcore_verbose=false  block_type=cic_compiler_v3_0
  Error Analysis : Subsystem
  Gain : Subsystem
  Gain1 : Subsystem
  Gain2 : Subsystem
  Gain3 : Subsystem
  Goto Tag Visibility : GotoTagVisibility  GotoTag=FOFB_FPGA_X_OUT
  Goto Tag Visibility1 : GotoTagVisibility  GotoTag=MONIT_CIC_X_FPGA_OUT
  Goto Tag Visibility10 : GotoTagVisibility  GotoTag=MONIT_CFIR_Q_FPGA_OUT
  Goto Tag Visibility11 : GotoTagVisibility  GotoTag=MONIT_PFIR_Q_FPGA_OUT
  Goto Tag Visibility12 : GotoTagVisibility  GotoTag=MONIT_CFIR_SUM_FPGA_OUT
  Goto Tag Visibility13 : GotoTagVisibility  GotoTag=MONIT_PFIR_SUM_FPGA_OUT
  Goto Tag Visibility14 : GotoTagVisibility  GotoTag=FOFB_FPGA_SUM_OUT
  Goto Tag Visibility15 : GotoTagVisibility  GotoTag=MONIT_CIC_SUM_FPGA_OUT
  Goto Tag Visibility2 : GotoTagVisibility  GotoTag=FOFB_FPGA_Y_OUT
  Goto Tag Visibility3 : GotoTagVisibility  GotoTag=MONIT_CIC_Y_FPGA_OUT
  Goto Tag Visibility4 : GotoTagVisibility  GotoTag=MONIT_CFIR_Y_FPGA_OUT
  Goto Tag Visibility5 : GotoTagVisibility  GotoTag=MONIT_CFIR_X_FPGA_OUT
  Goto Tag Visibility6 : GotoTagVisibility  GotoTag=MONIT_PFIR_X_FPGA_OUT
  Goto Tag Visibility7 : GotoTagVisibility  GotoTag=MONIT_PFIR_Y_FPGA_OUT
  Goto Tag Visibility8 : GotoTagVisibility  GotoTag=FOFB_FPGA_Q_OUT
  Goto Tag Visibility9 : GotoTagVisibility  GotoTag=MONIT_CIC_Q_FPGA_OUT
  PFIR_monit : xbsIndex_r4/FIR Compiler 6.3   coefficientvector=hpfir_sec.Numerator  coefficient_sets=1  coefficient_reload=off  filter_type=Decimation  rate_change_type=Integer  interpolation_rate=1  decimation_rate=2  zero_pack_factor=1  channel_sequence=Basic  number_channels=1  pattern_list='P4-0,P4-1,P4-2,P4-3,P4-4'  number_paths=4  ratespecification=Hardware_Oversampling_Rate  sampleperiod=5565000  hardwareoversamplingrate=1  coefficient_sign=Signed  quantization=Integer_Coefficients  coefficient_width=16  bestprecision=off  coefficient_fractional_bits=0  coefficient_structure=Inferred  output_rounding_mode=Full_Precision  output_width=34  filter_architecture=Systolic_Multiply_Accumulate  optimization_goal=Area  data_buffer_type=Automatic  coefficient_buffer_type=Automatic  input_buffer_type=Automatic  output_buffer_type=Automatic  preference_for_other_storage=Automatic  multi_column_support=Automatic  columnconfig='21'  inter_column_pipe_length=4  data_has_tlast=Not_Required  m_data_has_tready=off  s_data_has_fifo=off  s_data_has_tuser=Not_Required  m_data_has_tuser=Not_Required  s_config_sync_mode=On_Vector  s_config_method=Single  num_reload_slots=1  has_aclken=off  has_aresetn=off  infoeditControl=ARESETn must be asserted for a minmum of 2 cycles  trim_axipin_name=on  passband_min=0.0  passband_max=0.5  stopband_min=0.5  stopband_max=1.0  filter_selection=1  gui_behaviour=Sysgen_GUI  data_sign=Signed  data_width=16  data_fractional_bits=0  data_tuser_width=1  wrapper_available=true  ip_wrap_arbitrary_binary_point=true  simulation_type=external_xfix  simulation_model=firv6_3_CModel:firv6_3_cmodel  ip_name=FIR Compiler  ip_version=6.3  dsptool_ready=true  ipcore_usecache=true  ipcore_useipmodelcache=true  ipcore_xco_need_fpga_part=true  port_translation_map={ 'aclken' => 'en', 'aresetn' => 'rst' }  run_core_at_system_period=true  ipcore_fpga_part=xlipgetpartsetting(gcb, {'virtex6', 'xc6vlx75t', '-3', 'ff784'})  block_type=fir_compiler_v6_3
      settings: infoedit=Maximum Possible : Maximizes oversampling rate. Abstracted input handshake (no s_data_tvalid) and automatic rate propagation.<br>Hardware Oversampling Rate : Specifies oversampling rate relative to the input sample period. Abstracted input handshake (no s_data_tvalid) and automatic rate propagation.<br>Sample Period : Specifies absolute oversampling rate. No input handshake abstraction (exposes s_data_tvalid) and no rate propagation.
  Reg : Subsystem
  Reg1 : Subsystem
  Reg2 : Subsystem
  Reg3 : Subsystem
  Round1 : Subsystem
  Round2 : Subsystem
  Round3 : Subsystem
  Round4 : Subsystem
  ST1 : Subsystem
  ST2 : Subsystem
  ST3 : Subsystem
  ST4 : Subsystem
  ST5 : Subsystem
  ST6 : Subsystem
  Terminator{,1..5,7..12} (12 alike) : Terminator
  y_monit_cfir_o : xbsIndex_r4/Gateway Out  inherit_from_input=on  hdl_port=on  timing_constraint=None  locs_specified=off  LOCs={}  UseAsDAC=off  DACChannel='1'  block_type=gatewayout
      settings: infoedit="Gateway out block.  Converts Xilinx fixed-point or floating-point type inputs into ouputs of type Simulink integer, single, double, or fixed point.<br><br>Hardware notes:  In hardware these blocks become top level output ports or are discarded, depending on how they are configured."
  y_monit_cfir_trunc_o : xbsIndex_r4/Gateway Out  inherit_from_input=on  hdl_port=on  timing_constraint=None  locs_specified=off  LOCs={}  UseAsDAC=off  DACChannel='1'  block_type=gatewayout
      settings: infoedit="Gateway out block.  Converts Xilinx fixed-point or floating-point type inputs into ouputs of type Simulink integer, single, double, or fixed point.<br><br>Hardware notes:  In hardware these blocks become top level output ports or are discarded, depending on how they are configured."
  y_monit_cic_o : xbsIndex_r4/Gateway Out  inherit_from_input=on  hdl_port=on  timing_constraint=None  locs_specified=off  LOCs={}  UseAsDAC=off  DACChannel='1'  block_type=gatewayout
      settings: infoedit="Gateway out block.  Converts Xilinx fixed-point or floating-point type inputs into ouputs of type Simulink integer, single, double, or fixed point.<br><br>Hardware notes:  In hardware these blocks become top level output ports or are discarded, depending on how they are configured."
  y_monit_cic_trunc_o : xbsIndex_r4/Gateway Out  inherit_from_input=on  hdl_port=on  timing_constraint=None  locs_specified=off  LOCs={}  UseAsDAC=off  DACChannel='1'  block_type=gatewayout
      settings: infoedit="Gateway out block.  Converts Xilinx fixed-point or floating-point type inputs into ouputs of type Simulink integer, single, double, or fixed point.<br><br>Hardware notes:  In hardware these blocks become top level output ports or are discarded, depending on how they are configured."
  y_monit_pfir_gain_o : xbsIndex_r4/Gateway Out  inherit_from_input=on  hdl_port=on  timing_constraint=None  locs_specified=off  LOCs={}  UseAsDAC=off  DACChannel='1'  block_type=gatewayout
      settings: infoedit="Gateway out block.  Converts Xilinx fixed-point or floating-point type inputs into ouputs of type Simulink integer, single, double, or fixed point.<br><br>Hardware notes:  In hardware these blocks become top level output ports or are discarded, depending on how they are configured."
  y_monit_pfir_o : xbsIndex_r4/Gateway Out  inherit_from_input=on  hdl_port=on  timing_constraint=None  locs_specified=off  LOCs={}  UseAsDAC=off  DACChannel='1'  block_type=gatewayout
      settings: infoedit="Gateway out block.  Converts Xilinx fixed-point or floating-point type inputs into ouputs of type Simulink integer, single, double, or fixed point.<br><br>Hardware notes:  In hardware these blocks become top level output ports or are discarded, depending on how they are configured."
  Monit_X_Out : Outport
  Monit_Valid_X_out : Outport  Port=2
  Monit_Y_Out : Outport  Port=3
  Monit_Valid_Y_out : Outport  Port=4
  Monit_Q_Out : Outport  Port=5
  Monit_Valid_Q_out : Outport  Port=6
  Monit_Sum_Out : Outport  Port=7
  Monit_Valid_Sum_out : Outport  Port=8
  tag scope: FOFB_FPGA_Q_OUT=scoped, FOFB_FPGA_SUM_OUT=scoped, FOFB_FPGA_X_OUT=scoped, FOFB_FPGA_Y_OUT=scoped, MONIT_CFIR_Q_FPGA_OUT=scoped, MONIT_CFIR_SUM_FPGA_OUT=scoped, MONIT_CFIR_X_FPGA_OUT=scoped, MONIT_CFIR_Y_FPGA_OUT=scoped, MONIT_CIC_Q_FPGA_OUT=scoped, MONIT_CIC_SUM_FPGA_OUT=scoped, MONIT_CIC_X_FPGA_OUT=scoped, MONIT_CIC_Y_FPGA_OUT=scoped, MONIT_PFIR_Q_FPGA_OUT=scoped, MONIT_PFIR_SUM_FPGA_OUT=scoped, MONIT_PFIR_X_FPGA_OUT=scoped, MONIT_PFIR_Y_FPGA_OUT=scoped
  wires:
  CIC_monit_X/1 -> Terminator3/1
  Round4/1(out) -> [MONIT_CFIR_X_FPGA_OUT], PFIR_monit/1
  Reg/1(out) -> [MONIT_CIC_X_FPGA_OUT], CFIR_monit/1
  CIC_monit_X/3 -> Reg/1(data_in)
  Data_in_X/1 -> CIC_monit_X/1, [FOFB_FPGA_X_OUT]
  CIC_monit_X/2 -> Reg/2(en)
  Gain/1(data_out) -> Monit_X_Out/1, [MONIT_PFIR_X_FPGA_OUT]
  Gain/2(valid) -> Monit_Valid_X_out/1
  CIC_monit_Y/1 -> Terminator2/1
  Data_in_Y/1 -> CIC_monit_Y/1, [FOFB_FPGA_Y_OUT]
  Data_in_Q/1 -> CIC_monit_Q/1, [FOFB_FPGA_Q_OUT]
  Reg1/1(out) -> CFIR_monit/2, [MONIT_CIC_Y_FPGA_OUT], ST2/1(In), y_monit_cic_trunc_o/1
  CIC_monit_Y/3 -> Reg1/1(data_in), y_monit_cic_o/1
  CIC_monit_Y/2 -> Reg1/2(en)
  Reg2/1(out) -> [MONIT_CIC_Q_FPGA_OUT], CFIR_monit/3
  CIC_monit_Q/3 -> Reg2/1(data_in)
  CIC_monit_Q/2 -> Reg2/2(en)
  Round1/1(out) -> [MONIT_CFIR_Y_FPGA_OUT], PFIR_monit/2, ST1/1(In), y_monit_cfir_trunc_o/1
  Round2/1(out) -> [MONIT_CFIR_Q_FPGA_OUT], PFIR_monit/3
  Gain1/1(data_out) -> [MONIT_PFIR_Y_FPGA_OUT], Monit_Y_Out/1, ST6/1(In), y_monit_pfir_gain_o/1
  Gain1/2(valid) -> Monit_Valid_Y_out/1
  Gain2/1(data_out) -> Monit_Q_Out/1, [MONIT_PFIR_Q_FPGA_OUT]
  Gain2/2(valid) -> Monit_Valid_Q_out/1
  Data_in_Sum/1 -> [FOFB_FPGA_SUM_OUT], CIC_monit_Sum/1
  Reg3/1(out) -> [MONIT_CIC_SUM_FPGA_OUT], CFIR_monit/4
  CIC_monit_Sum/3 -> Reg3/1(data_in)
  CIC_monit_Sum/2 -> Reg3/2(en)
  Round3/1(out) -> [MONIT_CFIR_SUM_FPGA_OUT], PFIR_monit/4
  CFIR_monit/6 -> Round3/1(data_in)
  CFIR_monit/5 -> Round2/1(data_in)
  CFIR_monit/4 -> ST3/1(In), Round1/1(data_in), y_monit_cfir_o/1
  CFIR_monit/3 -> ST4/1(In), Round4/1(data_in)
  CFIR_monit/2 -> Round2/2(en), Round3/2(en), Round1/2(en), Round4/2(en)
  Gain3/1(data_out) -> Monit_Sum_Out/1, [MONIT_PFIR_SUM_FPGA_OUT]
  Gain3/2(valid) -> Monit_Valid_Sum_out/1
  PFIR_monit/3 -> Gain/1(data_in)
  PFIR_monit/4 -> ST5/1(In), Gain1/1(data_in), y_monit_pfir_o/1
  PFIR_monit/5 -> Gain2/1(data_in)
  PFIR_monit/6 -> Gain3/1(data_in)
  PFIR_monit/2 -> Gain2/2(en), Gain3/2(en), Gain1/2(en), Gain/2(en)
  CFIR_monit/1 -> Terminator/1
  CIC_monit_Sum/1 -> Terminator1/1
  PFIR_monit/1 -> Terminator5/1
  CIC_monit_Q/1 -> Terminator4/1
  y_monit_cfir_o/1 -> Terminator7/1
  y_monit_cfir_trunc_o/1 -> Terminator8/1
  y_monit_cic_o/1 -> Terminator9/1
  y_monit_cic_trunc_o/1 -> Terminator10/1
  y_monit_pfir_gain_o/1 -> Terminator11/1
  y_monit_pfir_o/1 -> Terminator12/1

== system ddc_bpm_476_066/ST1 ==
  In : Inport
  Display : Display
  Sample Time : xbsIndex_r4/Sample Time  block_type=sampletime
      settings: infoedit="The Sample Time block reports the normalized sample period of its input.  A signal's normalized sample period is not equivalent to its Simulink absolute sample period.<br><br>Hardware notes: This block is implemented as a constant in hardware."
  X_monit1 : xbsIndex_r4/Gateway Out  inherit_from_input=on  hdl_port=off  timing_constraint=Data Rate  locs_specified=off  LOCs={}  UseAsDAC=off  DACChannel='1'  block_type=gatewayout
      settings: infoedit="Gateway out block.  Converts Xilinx fixed-point or floating-point type inputs into ouputs of type Simulink integer, single, double, or fixed point.<br><br>Hardware notes:  In hardware these blocks become top level output ports or are discarded, depending on how they are configured."
  wires:
  X_monit1/1 -> Display/1
  Sample Time/1 -> X_monit1/1
  In/1 -> Sample Time/1

== system ddc_bpm_476_066/ST2 ==
  In : Inport
  Display : Display
  Sample Time : xbsIndex_r4/Sample Time  block_type=sampletime
      settings: infoedit="The Sample Time block reports the normalized sample period of its input.  A signal's normalized sample period is not equivalent to its Simulink absolute sample period.<br><br>Hardware notes: This block is implemented as a constant in hardware."
  X_monit1 : xbsIndex_r4/Gateway Out  inherit_from_input=on  hdl_port=off  timing_constraint=Data Rate  locs_specified=off  LOCs={}  UseAsDAC=off  DACChannel='1'  block_type=gatewayout
      settings: infoedit="Gateway out block.  Converts Xilinx fixed-point or floating-point type inputs into ouputs of type Simulink integer, single, double, or fixed point.<br><br>Hardware notes:  In hardware these blocks become top level output ports or are discarded, depending on how they are configured."
  wires:
  X_monit1/1 -> Display/1
  Sample Time/1 -> X_monit1/1
  In/1 -> Sample Time/1
